simulink model "scdskyhogg"  (Simulink 7.6)
settings: Solver=ode45  StartTime=0.0  StopTime=75  RelTol=1e-3
model workspace (MAT data in the model file):
  cg_0 = [2.158 0 0]
  g_0 = [0 0 9.81]
  Sref = 20.9775
  bref = 12.5425
  cbar = 1.7526
  Thrust = 2512.574
  maxdef_aileron = 30
  mindef_aileron = -30
  maxdef_elevator = 20
  mindef_elevator = -20
  maxdef_rudder = 60
  mindef_rudder = -60
  wn_act = 44
  z_act = 0.7
  LatLong0 = [45 120]
  heading0 = 0
  Tc = 0.0166666666667
  mass = 1299.21378662
  inertia = [5787.969  0  117.64; 0  6928.93  0; -117.64  0  11578.329]
  Ts = 0
  alpha0 = 0.0170924
  V0 = 93.1047999839
  beta0 = 0
  alt0 = 2000
  wy0 = 0
  theta0 = 0.017092
  mpoperpoint : opcond.OperatingPoint (value not decoded)
  op : opcond.OperatingPoint (value not decoded)
  x0.time = 75
  x0.signals(1).values = 0
  x0.signals(1).dimensions = 1
  x0.signals(1).label = 'CSTATE'
  x0.signals(1).blockName = 'scdskyhogg/Environment/Wind Models/Discrete Wind Gust Model/Distance into
    | gust (x)/Distance into
    | Gust (x)
    | (Limited to gust length d)'
  x0.signals(1).stateName = ''
  x0.signals(1).inReferencedModel = 0
  x0.signals(1).sampleTime = [0 0]
  x0.signals(2).values = 0
  x0.signals(2).dimensions = 1
  x0.signals(2).label = 'CSTATE'
  x0.signals(2).blockName = 'scdskyhogg/Environment/Wind Models/Discrete Wind Gust Model/Distance into
    | gust (y)/Distance into
    | Gust (x)
    | (Limited to gust length d)
    | '
  x0.signals(2).stateName = ''
  x0.signals(2).inReferencedModel = 0
  x0.signals(2).sampleTime = [0 0]
  x0.signals(3).values = 0
  x0.signals(3).dimensions = 1
  x0.signals(3).label = 'CSTATE'
  x0.signals(3).blockName = 'scdskyhogg/Environment/Wind Models/Discrete Wind Gust Model/Distance into
    | gust (z)/Distance into
    | Gust (x)
    | (Limited to gust length d)
    | '
  x0.signals(3).stateName = ''
  x0.signals(3).inReferencedModel = 0
  x0.signals(3).sampleTime = [0 0]
  x0.signals(4).values = [0 0]
  x0.signals(4).dimensions = 2
  x0.signals(4).label = 'CSTATE'
  x0.signals(4).blockName = 'scdskyhogg/Environment/Wind Models/Dryden Wind Turbulence Model 
    | (Continuous (+q +r))/Filters on angular rates/Hpgw/pgw_p'
  x0.signals(4).stateName = ''
  x0.signals(4).inReferencedModel = 0
  x0.signals(4).sampleTime = [0 0]
  x0.signals(5).values = [0 0]
  x0.signals(5).dimensions = 2
  x0.signals(5).label = 'CSTATE'
  x0.signals(5).blockName = 'scdskyhogg/Environment/Wind Models/Dryden Wind Turbulence Model 
    | (Continuous (+q +r))/Filters on angular rates/Hqgw/qgw_p'
  x0.signals(5).stateName = ''
  x0.signals(5).inReferencedModel = 0
  x0.signals(5).sampleTime = [0 0]
  x0.signals(6).values = [0 0]
  x0.signals(6).dimensions = 2
  x0.signals(6).label = 'CSTATE'
  x0.signals(6).blockName = 'scdskyhogg/Environment/Wind Models/Dryden Wind Turbulence Model 
    | (Continuous (+q +r))/Filters on angular rates/Hrgw/rgw_p'
  x0.signals(6).stateName = ''
  x0.signals(6).inReferencedModel = 0
  x0.signals(6).sampleTime = [0 0]
  x0.signals(7).values = [0 0]
  x0.signals(7).dimensions = 2
  x0.signals(7).label = 'CSTATE'
  x0.signals(7).blockName = 'scdskyhogg/Environment/Wind Models/Dryden Wind Turbulence Model 
    | (Continuous (+q +r))/Filters on velocities/Hugw(s)/ug_p'
  x0.signals(7).stateName = ''
  x0.signals(7).inReferencedModel = 0
  x0.signals(7).sampleTime = [0 0]
  x0.signals(8).values = [0 0]
  x0.signals(8).dimensions = 2
  x0.signals(8).label = 'CSTATE'
  x0.signals(8).blockName = 'scdskyhogg/Environment/Wind Models/Dryden Wind Turbulence Model 
    | (Continuous (+q +r))/Filters on velocities/Hvgw(s)/vg_p1'
  x0.signals(8).stateName = ''
  x0.signals(8).inReferencedModel = 0
  x0.signals(8).sampleTime = [0 0]
  x0.signals(9).values = [0 0]
  x0.signals(9).dimensions = 2
  x0.signals(9).label = 'CSTATE'
  x0.signals(9).blockName = 'scdskyhogg/Environment/Wind Models/Dryden Wind Turbulence Model 
    | (Continuous (+q +r))/Filters on velocities/Hvgw(s)/vgw_p2'
  x0.signals(9).stateName = ''
  x0.signals(9).inReferencedModel = 0
  x0.signals(9).sampleTime = [0 0]
  x0.signals(10).values = [0 0]
  x0.signals(10).dimensions = 2
  x0.signals(10).label = 'CSTATE'
  x0.signals(10).blockName = 'scdskyhogg/Environment/Wind Models/Dryden Wind Turbulence Model 
    | (Continuous (+q +r))/Filters on velocities/Hwgw(s)/wg_p1'
  x0.signals(10).stateName = ''
  x0.signals(10).inReferencedModel = 0
  x0.signals(10).sampleTime = [0 0]
  x0.signals(11).values = [0 0]
  x0.signals(11).dimensions = 2
  x0.signals(11).label = 'CSTATE'
  x0.signals(11).blockName = 'scdskyhogg/Environment/Wind Models/Dryden Wind Turbulence Model 
    | (Continuous (+q +r))/Filters on velocities/Hwgw(s)/wg_p2'
  x0.signals(11).stateName = ''
  x0.signals(11).inReferencedModel = 0
  x0.signals(11).sampleTime = [0 0]
  x0.signals(12).values = 8000
  x0.signals(12).dimensions = 1
  x0.signals(12).label = 'CSTATE'
  x0.signals(12).blockName = 'scdskyhogg/Pilot/Transfer Fcn
    | (with initial outputs)/State Space'
  x0.signals(12).stateName = ''
  x0.signals(12).inReferencedModel = 0
  x0.signals(12).sampleTime = [0 0]
  x0.signals(13).values = [19554.3139246 18764.5538786]
  x0.signals(13).dimensions = 2
  x0.signals(13).label = 'DSTATE'
  x0.signals(13).blockName = 'scdskyhogg/Vehicle System Model/Avionics/Autopilot/Alt Controller'
  x0.signals(13).stateName = ''
  x0.signals(13).inReferencedModel = 0
  x0.signals(13).sampleTime = [0.0166666666667 0]
  x0.signals(14).values = 4.54490878098
  x0.signals(14).dimensions = 1
  x0.signals(14).label = 'DSTATE'
  x0.signals(14).blockName = 'scdskyhogg/Vehicle System Model/Avionics/Autopilot/Theta Controller'
  x0.signals(14).stateName = ''
  x0.signals(14).inReferencedModel = 0
  x0.signals(14).sampleTime = [0.0166666666667 0]
  x0.signals(15).values = [0 0]
  x0.signals(15).dimensions = 2
  x0.signals(15).label = 'DSTATE'
  x0.signals(15).blockName = 'scdskyhogg/Vehicle System Model/Avionics/Three-axis IMU/Three-axis Accelerometer/Dynamics/Second-order Dynamics/Transfer Fcn X/Discrete
    | Transfer Fcn'
  x0.signals(15).stateName = ''
  x0.signals(15).inReferencedModel = 0
  x0.signals(15).sampleTime = [0.0166666666667 0]
  x0.signals(16).values = [0 0]
  x0.signals(16).dimensions = 2
  x0.signals(16).label = 'DSTATE'
  x0.signals(16).blockName = 'scdskyhogg/Vehicle System Model/Avionics/Three-axis IMU/Three-axis Accelerometer/Dynamics/Second-order Dynamics/Transfer Fcn Y/Discrete
    | Transfer Fcn'
  x0.signals(16).stateName = ''
  x0.signals(16).inReferencedModel = 0
  x0.signals(16).sampleTime = [0.0166666666667 0]
  x0.signals(17).values = [0 0]
  x0.signals(17).dimensions = 2
  x0.signals(17).label = 'DSTATE'
  x0.signals(17).blockName = 'scdskyhogg/Vehicle System Model/Avionics/Three-axis IMU/Three-axis Accelerometer/Dynamics/Second-order Dynamics/Transfer Fcn Z/Discrete
    | Transfer Fcn'
  x0.signals(17).stateName = ''
  x0.signals(17).inReferencedModel = 0
  x0.signals(17).sampleTime = [0.0166666666667 0]
  x0.signals(18).values = [0 0]
  x0.signals(18).dimensions = 2
  x0.signals(18).label = 'DSTATE'
  x0.signals(18).blockName = 'scdskyhogg/Vehicle System Model/Avionics/Three-axis IMU/Three-axis Gyroscope/Dynamics/Second-order Dynamics/Transfer Fcn X/Discrete
    | Transfer Fcn'
  x0.signals(18).stateName = ''
  x0.signals(18).inReferencedModel = 0
  x0.signals(18).sampleTime = [0.0166666666667 0]
  x0.signals(19).values = [0 0]
  x0.signals(19).dimensions = 2
  x0.signals(19).label = 'DSTATE'
  x0.signals(19).blockName = 'scdskyhogg/Vehicle System Model/Avionics/Three-axis IMU/Three-axis Gyroscope/Dynamics/Second-order Dynamics/Transfer Fcn Y/Discrete
    | Transfer Fcn'
  x0.signals(19).stateName = ''
  x0.signals(19).inReferencedModel = 0
  x0.signals(19).sampleTime = [0.0166666666667 0]
  x0.signals(20).values = [0 0]
  x0.signals(20).dimensions = 2
  x0.signals(20).label = 'DSTATE'
  x0.signals(20).blockName = 'scdskyhogg/Vehicle System Model/Avionics/Three-axis IMU/Three-axis Gyroscope/Dynamics/Second-order Dynamics/Transfer Fcn Z/Discrete
    | Transfer Fcn'
  x0.signals(20).stateName = ''
  x0.signals(20).inReferencedModel = 0
  x0.signals(20).sampleTime = [0.0166666666667 0]
  x0.signals(21).values = [6983.69332589 -2000.01117817]
  x0.signals(21).dimensions = 2
  x0.signals(21).label = 'CSTATE'
  x0.signals(21).blockName = 'scdskyhogg/Vehicle System Model/Vehicle/3DoF to 6DoF/3DoF (Body Axes)/Position'
  x0.signals(21).stateName = ''
  x0.signals(21).inReferencedModel = 0
  x0.signals(21).sampleTime = [0 0]
  x0.signals(22).values = 0.0170954076892
  x0.signals(22).dimensions = 1
  x0.signals(22).label = 'CSTATE'
  x0.signals(22).blockName = 'scdskyhogg/Vehicle System Model/Vehicle/3DoF to 6DoF/3DoF (Body Axes)/Theta'
  x0.signals(22).stateName = ''
  x0.signals(22).inReferencedModel = 0
  x0.signals(22).sampleTime = [0 0]
  x0.signals(23).values = [93.0805745614 1.59150213219]
  x0.signals(23).dimensions = 2
  x0.signals(23).label = 'CSTATE'
  x0.signals(23).blockName = 'scdskyhogg/Vehicle System Model/Vehicle/3DoF to 6DoF/3DoF (Body Axes)/U,w'
  x0.signals(23).stateName = ''
  x0.signals(23).inReferencedModel = 0
  x0.signals(23).sampleTime = [0 0]
  x0.signals(24).values = -4.21452165535e-07
  x0.signals(24).dimensions = 1
  x0.signals(24).label = 'CSTATE'
  x0.signals(24).blockName = 'scdskyhogg/Vehicle System Model/Vehicle/3DoF to 6DoF/3DoF (Body Axes)/q'
  x0.signals(24).stateName = ''
  x0.signals(24).inReferencedModel = 0
  x0.signals(24).sampleTime = [0 0]
  x0.signals(25).values = 0
  x0.signals(25).dimensions = 1
  x0.signals(25).label = 'CSTATE'
  x0.signals(25).blockName = 'scdskyhogg/Vehicle System Model/Vehicle/AirframeActuators/2nd Order Non-linear Actuator/Limited
    | Deflection'
  x0.signals(25).stateName = ''
  x0.signals(25).inReferencedModel = 0
  x0.signals(25).sampleTime = [0 0]
  x0.signals(26).values = 0
  x0.signals(26).dimensions = 1
  x0.signals(26).label = 'CSTATE'
  x0.signals(26).blockName = 'scdskyhogg/Vehicle System Model/Vehicle/AirframeActuators/2nd Order Non-linear Actuator/Servo rate'
  x0.signals(26).stateName = ''
  x0.signals(26).inReferencedModel = 0
  x0.signals(26).sampleTime = [0 0]
  x0.signals(27).values = -0.905026907299
  x0.signals(27).dimensions = 1
  x0.signals(27).label = 'CSTATE'
  x0.signals(27).blockName = 'scdskyhogg/Vehicle System Model/Vehicle/AirframeActuators/2nd Order Non-linear Actuator1/Limited
    | Deflection'
  x0.signals(27).stateName = ''
  x0.signals(27).inReferencedModel = 0
  x0.signals(27).sampleTime = [0 0]
  x0.signals(28).values = 7.66583857879e-05
  x0.signals(28).dimensions = 1
  x0.signals(28).label = 'CSTATE'
  x0.signals(28).blockName = 'scdskyhogg/Vehicle System Model/Vehicle/AirframeActuators/2nd Order Non-linear Actuator1/Servo rate'
  x0.signals(28).stateName = ''
  x0.signals(28).inReferencedModel = 0
  x0.signals(28).sampleTime = [0 0]
  x0.signals(29).values = 0
  x0.signals(29).dimensions = 1
  x0.signals(29).label = 'CSTATE'
  x0.signals(29).blockName = 'scdskyhogg/Vehicle System Model/Vehicle/AirframeActuators/2nd Order Non-linear Actuator2/Limited
    | Deflection'
  x0.signals(29).stateName = ''
  x0.signals(29).inReferencedModel = 0
  x0.signals(29).sampleTime = [0 0]
  x0.signals(30).values = 0
  x0.signals(30).dimensions = 1
  x0.signals(30).label = 'CSTATE'
  x0.signals(30).blockName = 'scdskyhogg/Vehicle System Model/Vehicle/AirframeActuators/2nd Order Non-linear Actuator2/Servo rate'
  x0.signals(30).stateName = ''
  x0.signals(30).inReferencedModel = 0
  x0.signals(30).sampleTime = [0 0]
PreLoadFcn:
  | load asbSkyHoggData.mat
StartFcn:
  | warning('off','Simulink:blocks:BmathSqrtOfNegativeNumber');
  | warning('off','Simulink:Engine:UINotUpdatedDuringRapidAccelSim')
StopFcn:
  | warning('on','Simulink:blocks:BmathSqrtOfNegativeNumber');
values from neighbouring files (symbols this model uses):
  mass = 13.98/Kg2slug    (= 204.022661401)    [scd_aero_guid_dat.m]
  Tc = simout.time    [scdcompdelay_engspeed.m]
  Thrust = 10e3    (= 10000)    [scd_aero_guid_dat.m]
  Ts = 0.25    [scdcompdelay_engspeed.m]
undefined symbols (not defined in the file or in its folder): Earth, F, Light, MIL, statdyn, WGS84
libraries: aerolibasang x4, aerolibwind2 x3, aerolibtransform2 x3, aerolibactuator x3, aerolibatmos2 x2, aerolibobsolete x2, aerolibconvert2 x2, aerolibadyn x2, simulink x1, simulink_extras x1, aerolibnav x1, aerolib3dof2 x1
Description:
  | Lightweight Airplane Design
  | 
  | This is the three degree-of-freedom model of a lightweight four-seater
  | low wing monoplane with a longitudinal autopilot.
CloseFcn:
  | warning('on','Simulink:Engine:UINotUpdatedDuringRapidAccelSim')
settings Model: Creator=The MathWorks Inc.  SimulationMode=rapid-accelerator
settings DataIOCC: ExternalInput=[]  InitialState=x0  LoadExternalInput=on  LoadInitialState=on
settings OptimizationCC: InitFltsAndDblsToZero=on
settings DebuggingCC: AlgebraicLoopMsg=none  SaveWithParameterizedLinksMsg=none  SignalResolutionControl=TryResolveAllWithWarning  SolverPrmCheckMsg=none  UnconnectedInputMsg=none  UnconnectedOutputMsg=none  UnconnectedLineMsg=none  StrictBusMsg=Warning
settings GRTTargetCC: TargetFcnLib=ansi_tfl_tmw.mat

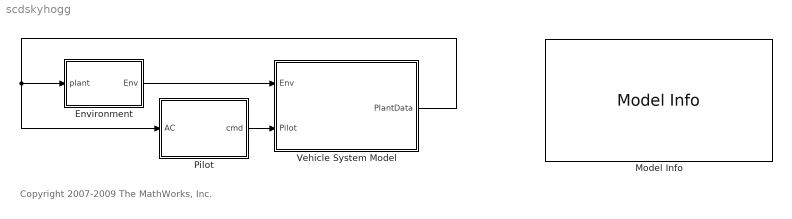
== system scdskyhogg ==
  note: Copyright 2007-2009 The MathWorks, Inc.
  Environment : Subsystem  TreatAsAtomicUnit=on
  Model Info : simulink/Model-Wide Utilities/Model Info  SystemSampleTime=-1  InitialBlockCM=None  BlockCM=None  Frame=on  DisplayStringWithTags=|  HorizontalTextAlignment=Center  LeftAlignmentValue=0.5  SourceBlockDiagram=scdskyhogg  TagMaxNumber=20
      | Sky Hogg demonstration model,
      | 
      | Vehicle Geometry from 
      | Cannon, M, Gabbard, M, Meyer, T, Morrison, 
      | S, Skocik, M, Woods, D. "Swineworks D-200 
      | Sky Hogg Design Proposal." AIAA/General 
      | Dynamics Corporation Team Aircraft Design
      |  Competition, 1991-1992
  Pilot : Subsystem  TreatAsAtomicUnit=on
  Vehicle System Model : Subsystem
      mask Display: image(imread('asbSkyHogg.jpg'),[.1 .1 .8 .8],'on')
  wires:
  Environment/1(Env) -> Vehicle System Model/1(Env)
  Vehicle System Model/1(PlantData) -> Environment/1(plant), Pilot/1(AC)
  Pilot/1(cmd) -> Vehicle System Model/2(Pilot)

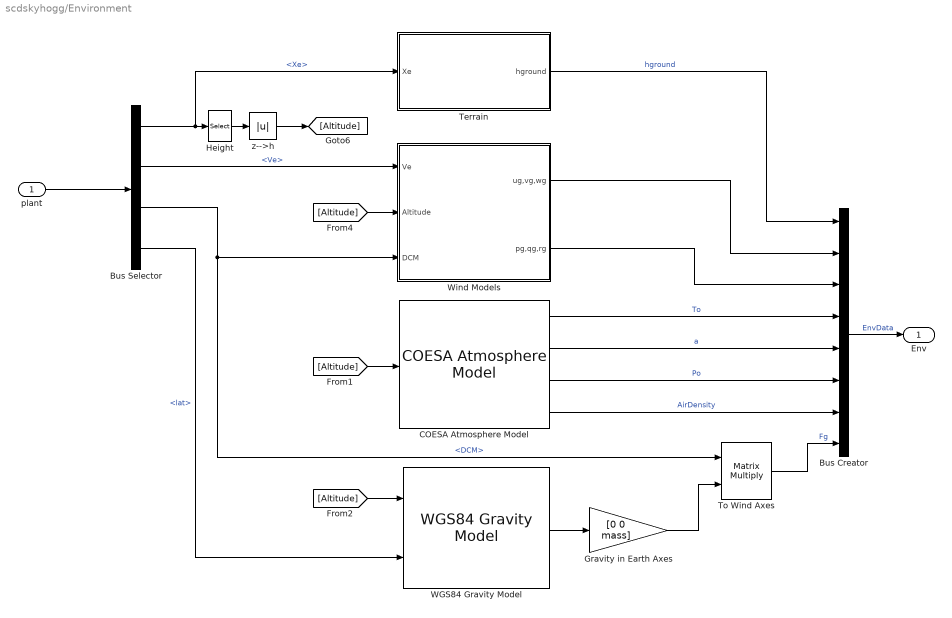
== system scdskyhogg/Environment ==
  plant : Inport
  Bus Creator : BusCreator  Inputs='hground','WindVelocity','WindAngularRates','To','a','Po','AirDensity','Fg'
  Bus Selector : BusSelector  OutputSignals=Xe,Ve,DCM,lat
  COESA Atmosphere Model : aerolibatmos2/COESA Atmosphere Model  SystemSampleTime=-1  units=Metric (MKS)  spec=1976 COESA-extended U.S. Standard Atmosphere  model=Profile  profile_var=High temperature  profile_percent=1%  profile_alt=5 km (16404 ft)  envelope_var=High temperature  envelope_percent=1%  action=Warning
  Gravity in Earth Axes : Gain  Gain=[0 0 mass]  SaturateOnIntegerOverflow=on  OutDataTypeStr=Inherit: Same as input  ParamDataTypeStr=Inherit: Same as input
  Height : Selector  InputPortWidth=3  IndexOptions=Index vector (dialog)  Indices=[3]  OutputSizes=1
  Terrain : Subsystem
  To Wind Axes : Product  Multiplication=Matrix(*)  SaturateOnIntegerOverflow=on  InputSameDT=on  OutDataTypeStr=Inherit: Same as first input
  WGS84 Gravity Model : aerolibobsolete/WGS84 Gravity Model  SystemSampleTime=-1  model=WGS84 Taylor Series  units=Metric (MKS)  no_atmos=on  precessing=on  month=February  day=1  year=2000  no_centrifugal=on  action=Warning
  Wind Models : Subsystem
  z-->h : Abs  SaturateOnIntegerOverflow=on
  Env : Outport  InitialOutput=0
  wires:
  Bus Selector/3 -> Wind Models/3(DCM), To Wind Axes/1  "<DCM>"
  Bus Selector/2 -> Wind Models/1(Ve)  "<Ve>"
  Bus Selector/1 -> Height/1, Terrain/1(Xe)  "<Xe>"
  [Altitude] -> COESA Atmosphere Model/1
  [Altitude] -> WGS84 Gravity Model/1
  [Altitude] -> Wind Models/2(Altitude)
  z-->h/1 -> [Altitude]
  plant/1 -> Bus Selector/1
  Bus Creator/1 -> Env/1  "EnvData"
  To Wind Axes/1 -> Bus Creator/8  "Fg"
  Gravity in Earth Axes/1 -> To Wind Axes/2
  WGS84 Gravity Model/1 -> Gravity in Earth Axes/1
  Bus Selector/4 -> WGS84 Gravity Model/2  "<lat>"
  Height/1 -> z-->h/1
  COESA Atmosphere Model/1 -> Bus Creator/4  "To"
  COESA Atmosphere Model/3 -> Bus Creator/6  "Po"
  COESA Atmosphere Model/2 -> Bus Creator/5  "a"
  COESA Atmosphere Model/4 -> Bus Creator/7  "AirDensity"
  Wind Models/2(pg,qg,rg) -> Bus Creator/3
  Wind Models/1(ug,vg,wg) -> Bus Creator/2
  Terrain/1(hground) -> Bus Creator/1  "hground"

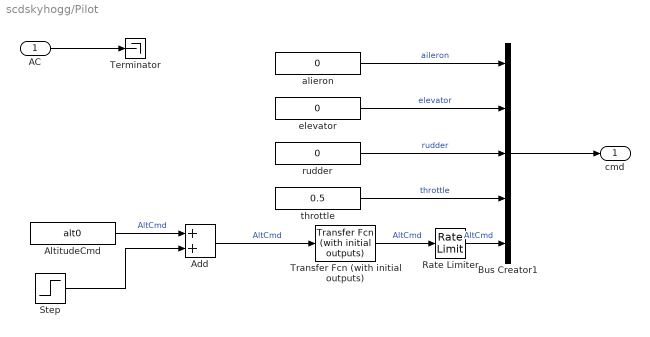
== system scdskyhogg/Pilot ==
  AC : Inport
  Add : Sum
  AltitudeCmd : Constant  Value=alt0  OutDataTypeStr=double
  Bus Creator1 : BusCreator  Inputs=5
  Rate Limiter : RateLimiter  RisingSlewLimit=500/3/60  SampleTimeMode=inherited  InitialCondition=2000
  Step : Step  Time=5  After=0  SampleTime=0
  Terminator : Terminator
  Transfer Fcn (with initial outputs) : simulink_extras/Additional Linear/Transfer Fcn (with initial outputs)  SystemSampleTime=-1  N=.25  D=[1,.25]  Y0=2000  U0=2000
  alieron : Constant  Value=0  OutDataTypeStr=single
  elevator : Constant  Value=0  OutDataTypeStr=single
  rudder : Constant  Value=0  OutDataTypeStr=single
  throttle : Constant  Value=0.5  OutDataTypeStr=double
  cmd : Outport
  wires:
  elevator/1 -> Bus Creator1/2  "elevator"
  alieron/1 -> Bus Creator1/1  "aileron"
  throttle/1 -> Bus Creator1/4  "throttle"
  rudder/1 -> Bus Creator1/3  "rudder"
  Bus Creator1/1 -> cmd/1
  AC/1 -> Terminator/1
  AltitudeCmd/1 -> Add/1  "AltCmd"
  Step/1 -> Add/2
  Add/1 -> Transfer Fcn (with initial outputs)/1  "AltCmd"
  Rate Limiter/1 -> Bus Creator1/5  "AltCmd"
  Transfer Fcn (with initial outputs)/1 -> Rate Limiter/1  "AltCmd"

== system scdskyhogg/Vehicle System Model ==
  Env : Inport
  Pilot : Inport  Port=2
  Avionics : Subsystem
  "Env " : InportShadow  Port=1
  Flight Sensors : Subsystem
  "Pilot " : InportShadow  Port=2
  Vehicle : Subsystem
  PlantData : Outport
  wires:
  Env/1 -> Vehicle/1(Env)
  Vehicle/1(PlantData) -> Avionics/1(PlantData), Flight Sensors/2(plant), PlantData/1
  Flight Sensors/1(sensed) -> Avionics/2(Sensors)
  Avionics/1(ActCmd) -> Vehicle/2(ActCmd)
  Pilot/1 -> Vehicle/3(Pilot)
  "Env "/1 -> Flight Sensors/1(Env)
  "Pilot "/1 -> Avionics/3(Pilot)

== system scdskyhogg/Environment/Terrain ==
  note: This part of the system defines the interface for the terrain model that will be developed in detail later on.
  Xe : Inport
  Terminator : Terminator
  hground_value : Constant  Value=0  OutDataTypeStr=single
  hground : Outport
  wires:
  hground_value/1 -> hground/1  "hground"
  Xe/1 -> Terminator/1

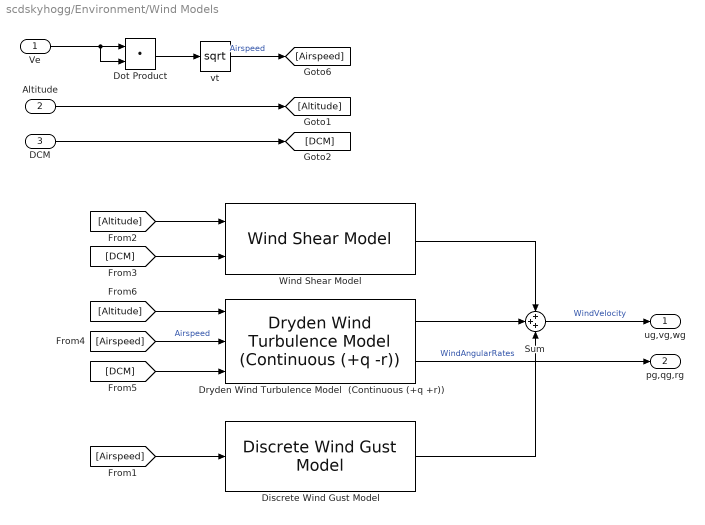
== system scdskyhogg/Environment/Wind Models ==
  Ve : Inport
  Altitude : Inport  Port=2
  DCM : Inport  Port=3
  Discrete Wind Gust Model : aerolibwind2/Discrete Wind Gust Model  SystemSampleTime=-1  units=Metric (MKS)  Gx=off  Gy=off  Gz=off  t_0=20  d_m=[120 120 80]  v_m=[3.5 3.0 3.0]
  Dot Product : DotProduct  OutDataTypeStr=Inherit: Inherit via internal rule
  Dryden Wind Turbulence Model  (Continuous (+q +r)) : aerolibwind2/Dryden Wind Turbulence Model  (Continuous (+q -r))  SystemSampleTime=-1  units=Metric (MKS)  spec=MIL-F-8785C  model=Continuous Dryden (+q +r)  W20=5  Wdeg=0  TurbProb=10^-2 - Light  L_high=533.4  Wingspan=4  ts=0.1  Seed=[23341 23342 23343 23344]  T_on=off
  Sum : Sum  Inputs=+++  SaturateOnIntegerOverflow=on  InputSameDT=on  OutDataTypeStr=Inherit: Same as first input
  Wind Shear Model : aerolibwind2/Wind Shear Model  SystemSampleTime=-1  units=Metric (MKS)  phase=Category C - Terminal Flight Phase  W_20=1  Wdeg=0
  vt : Math  Operator=sqrt  SaturateOnIntegerOverflow=on
  ug,vg,wg : Outport
  pg,qg,rg : Outport  Port=2
  wires:
  [Altitude] -> Dryden Wind Turbulence Model  (Continuous (+q +r))/1
  [DCM] -> Dryden Wind Turbulence Model  (Continuous (+q +r))/3
  [DCM] -> Wind Shear Model/2
  DCM/1 -> [DCM]
  [Altitude] -> Wind Shear Model/1
  Altitude/1 -> [Altitude]
  [Airspeed] -> Discrete Wind Gust Model/1
  vt/1 -> [Airspeed]  "Airspeed"
  Dot Product/1 -> vt/1
  Dryden Wind Turbulence Model  (Continuous (+q +r))/2 -> pg,qg,rg/1  "WindAngularRates"
  [Airspeed] -> Dryden Wind Turbulence Model  (Continuous (+q +r))/2  "Airspeed"
  Sum/1 -> ug,vg,wg/1  "WindVelocity"
  Discrete Wind Gust Model/1 -> Sum/3
  Dryden Wind Turbulence Model  (Continuous (+q +r))/1 -> Sum/2
  Wind Shear Model/1 -> Sum/1
  Ve/1 -> Dot Product/2, Dot Product/1

== system scdskyhogg/Vehicle System Model/Avionics ==
  PlantData : Inport
  Sensors : Inport  Port=2
  Pilot : Inport  Port=3
  Air Data Computer : Subsystem  TreatAsAtomicUnit=on
  Autopilot : Subsystem
  Bus Creator : BusCreator  Inputs=2
  Bus Selector1 : BusSelector  OutputSignals=Ab,w,wdot
  Center of Gravity : Constant  Value=cg_0  SampleTime=Tc
  Gravity (not in Accels) : Constant  Value=g_0  SampleTime=Tc
  Guidance : Subsystem
  Three-axis IMU : aerolibnav/Three-axis Inertial Measurement Unit  SystemSampleTime=-1  units=Metric (MKS)  imu=cg_0  dtype_a=off  w_a=190  z_a=0.707  a_sf_cc=[1 0 0; 0 1 0; 0 0 1]  a_bias=[0 0 0]  a_sat="[-inf  -inf  -inf  inf inf inf]"  dtype_g=off  w_g=190  z_g=0.707  g_sf_cc=[1 0 0; 0 1 0; 0 0 1]  g_bias=[0 0 0]  g_sens=[0 0 0]  g_sat="[-inf  -inf  -inf  inf inf inf]"  i_rand=off  i_seeds=[23093 23094 23095 23096 23097 23098]  i_pow=[0.001 0.001 0.001 0.0001 0.0001 0.0001]  i_Ts=Tc
  ActCmd : Outport
  wires:
  Three-axis IMU/2 -> Bus Creator/2
  Three-axis IMU/1 -> Bus Creator/1
  Bus Selector1/1 -> Three-axis IMU/1  "<Ab>"
  Center of Gravity/1 -> Three-axis IMU/4
  Bus Creator/1 -> Guidance/2(AvionicBus), Autopilot/1(AvionicBus)
  PlantData/1 -> Bus Selector1/1
  Bus Selector1/2 -> Three-axis IMU/2  "<w>"
  Bus Selector1/3 -> Three-axis IMU/3  "<wdot>"
  Gravity (not in Accels)/1 -> Three-axis IMU/5
  Sensors/1 -> Air Data Computer/1(sensors)
  Autopilot/1(cmd) -> ActCmd/1
  Air Data Computer/1(AirData) -> Guidance/1(AirData), Autopilot/2(AirData)
  Guidance/1(cmd) -> Autopilot/3(guidance)
  Pilot/1 -> Guidance/3(Pilot)

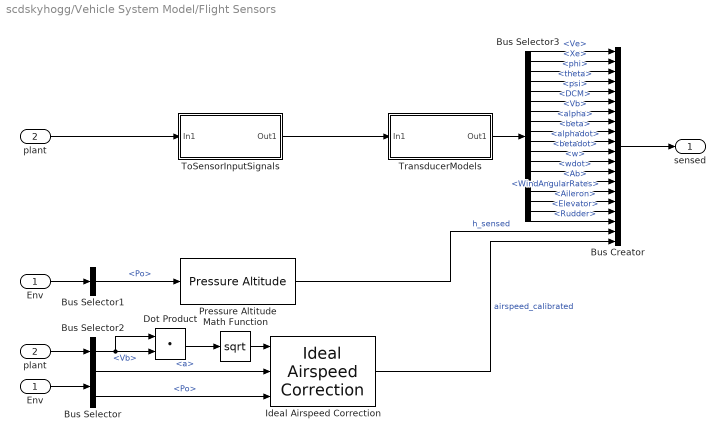
== system scdskyhogg/Vehicle System Model/Flight Sensors ==
  Env : Inport
  plant : Inport  Port=2
  Bus Creator : BusCreator  Inputs=20
  Bus Selector : BusSelector  OutputSignals=a,Po
  Bus Selector1 : BusSelector  OutputSignals=Po
  Bus Selector2 : BusSelector  OutputSignals=Vb
  Bus Selector3 : BusSelector  OutputSignals=Ve,Xe,body angles.phi,body angles.theta,body angles.psi,DCM,Vb,alpha,beta,alphadot,betadot,w,wdot,Ab,WindAngularRates,Act_positions.Aileron,Act_positions.Elevator,Act_positions.Rudder
  Dot Product : DotProduct  InputSameDT=on  OutDataTypeStr=Inherit: Inherit via internal rule
  "Env " : InportShadow  Port=1
  Ideal Airspeed Correction : aerolibasang/Ideal Airspeed Correction  SystemSampleTime=-1  units=Metric (MKS)  vel_in=TAS  vel_out_tas=CAS  vel_out_eas=CAS  vel_out_cas=TAS  action=Error
  Math Function : Math  Operator=sqrt  SaturateOnIntegerOverflow=on
  Pressure Altitude : aerolibatmos2/Pressure Altitude  SystemSampleTime=-1  units=Metric (MKS)  action=Warning
  ToSensorInputSignals : Subsystem
  TransducerModels : Subsystem
  "plant " : InportShadow  Port=2
  sensed : Outport
  wires:
  ToSensorInputSignals/1(Out1) -> TransducerModels/1(In1)
  Env/1 -> Bus Selector/1
  TransducerModels/1(Out1) -> Bus Selector3/1
  plant/1 -> ToSensorInputSignals/1(In1)
  Bus Selector/1 -> Ideal Airspeed Correction/2  "<a>"
  Bus Selector/2 -> Ideal Airspeed Correction/3  "<Po>"
  Bus Selector1/1 -> Pressure Altitude/1  "<Po>"
  "Env "/1 -> Bus Selector1/1
  "plant "/1 -> Bus Selector2/1
  Dot Product/1 -> Math Function/1
  Math Function/1 -> Ideal Airspeed Correction/1
  Bus Selector2/1 -> Dot Product/2, Dot Product/1  "<Vb>"
  Bus Selector3/1 -> Bus Creator/1  "<Ve>"
  Bus Selector3/2 -> Bus Creator/2  "<Xe>"
  Bus Selector3/3 -> Bus Creator/3  "<phi>"
  Bus Selector3/4 -> Bus Creator/4  "<theta>"
  Bus Selector3/5 -> Bus Creator/5  "<psi>"
  Bus Selector3/6 -> Bus Creator/6  "<DCM>"
  Bus Selector3/7 -> Bus Creator/7  "<Vb>"
  Bus Selector3/8 -> Bus Creator/8  "<alpha>"
  Bus Selector3/9 -> Bus Creator/9  "<beta>"
  Bus Selector3/10 -> Bus Creator/10  "<alphadot>"
  Bus Selector3/11 -> Bus Creator/11  "<betadot>"
  Bus Selector3/12 -> Bus Creator/12  "<w>"
  Bus Selector3/13 -> Bus Creator/13  "<wdot>"
  Bus Selector3/14 -> Bus Creator/14  "<Ab>"
  Bus Creator/1 -> sensed/1
  Bus Selector3/15 -> Bus Creator/15  "<WindAngularRates>"
  Bus Selector3/16 -> Bus Creator/16  "<Aileron>"
  Bus Selector3/17 -> Bus Creator/17  "<Elevator>"
  Bus Selector3/18 -> Bus Creator/18  "<Rudder>"
  Pressure Altitude/1 -> Bus Creator/19  "h_sensed"
  Ideal Airspeed Correction/1 -> Bus Creator/20  "airspeed_calibrated"

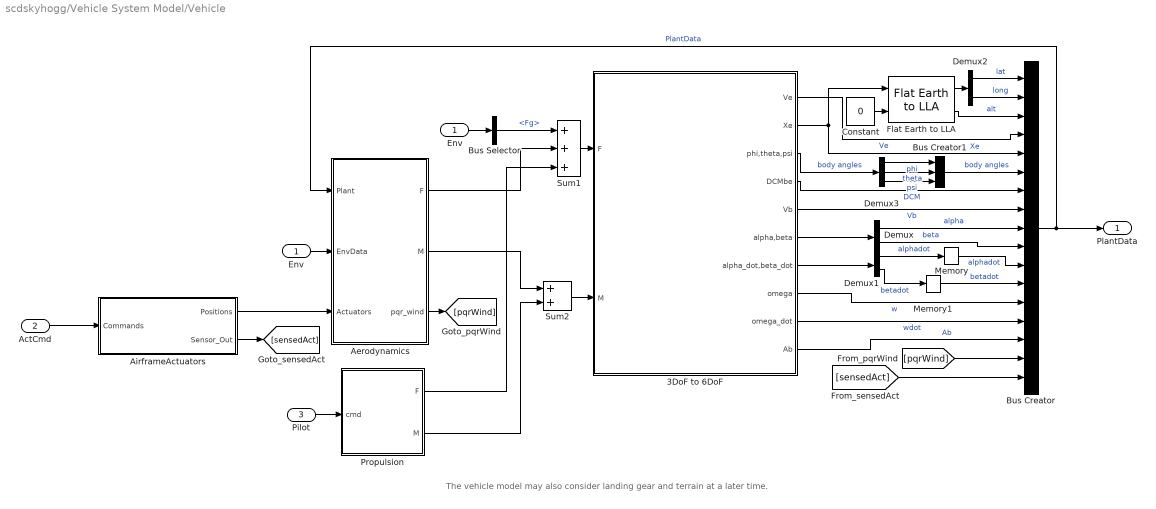
== system scdskyhogg/Vehicle System Model/Vehicle ==
  note: The vehicle model may also consider landing gear and terrain at a later time.
  Env : Inport
  ActCmd : Inport  Port=2
  Pilot : Inport  Port=3
  3DoF to 6DoF : Subsystem
  Aerodynamics : Subsystem
  AirframeActuators : Subsystem
  Bus Creator : BusCreator  Inputs=17
  Bus Creator1 : BusCreator  Inputs=3
  Bus Selector : BusSelector  OutputSignals=Fg
  Constant : Constant  Value=0
  Demux : Demux  Outputs=2
  Demux1 : Demux  Outputs=2
  Demux2 : Demux  Outputs=2
  Demux3 : Demux  Outputs=3
  "Env " : InportShadow  Port=1
  Flat Earth to LLA : aerolibtransform2/Flat Earth to LLA  SystemSampleTime=-1  units=Metric (MKS)  ptype=Earth (WGS84)  F=1/298.257223563  R=6378137  LL0=LatLong0  psi=heading0
  Memory : Memory  X0=alpha0  LinearizeMemory=on
  Memory1 : Memory  X0=beta0  LinearizeMemory=on
  Propulsion : Subsystem
      settings: RTWSystemCode=Inline
  Sum1 : Sum  Inputs=+++  SaturateOnIntegerOverflow=on  InputSameDT=on  OutDataTypeStr=Inherit: Same as first input
  Sum2 : Sum  SaturateOnIntegerOverflow=on  InputSameDT=on  OutDataTypeStr=Inherit: Same as first input
  PlantData : Outport
  wires:
  Sum1/1 -> 3DoF to 6DoF/1(F)
  Sum2/1 -> 3DoF to 6DoF/2(M)
  3DoF to 6DoF/3(phi,theta,psi) -> Demux3/1  "body angles"
  3DoF to 6DoF/4(DCMbe) -> Bus Creator/7  "DCM"
  3DoF to 6DoF/5(Vb) -> Bus Creator/8  "Vb"
  3DoF to 6DoF/6(alpha,beta) -> Demux/1
  3DoF to 6DoF/7(alpha_dot,beta_dot) -> Demux1/1
  3DoF to 6DoF/9(omega_dot) -> Bus Creator/14  "wdot"
  3DoF to 6DoF/10(Ab) -> Bus Creator/15  "Ab"
  Bus Creator/1 -> Aerodynamics/1(Plant), PlantData/1  "PlantData"
  Aerodynamics/1(F) -> Sum1/2
  Aerodynamics/2(M) -> Sum2/1
  Propulsion/1(F) -> Sum1/3
  Propulsion/2(M) -> Sum2/2
  Bus Selector/1 -> Sum1/1  "<Fg>"
  Env/1 -> Aerodynamics/2(EnvData)
  ActCmd/1 -> AirframeActuators/1(Commands)
  Pilot/1 -> Propulsion/1(cmd)
  "Env "/1 -> Bus Selector/1
  AirframeActuators/1(Positions) -> Aerodynamics/3(Actuators)
  Aerodynamics/3(pqr_wind) -> [pqrWind]
  [pqrWind] -> Bus Creator/16
  AirframeActuators/2(Sensor_Out) -> [sensedAct]
  [sensedAct] -> Bus Creator/17
  Constant/1 -> Flat Earth to LLA/2
  Flat Earth to LLA/2 -> Bus Creator/3  "alt"
  Flat Earth to LLA/1 -> Demux2/1
  Demux2/1 -> Bus Creator/1  "lat"
  Demux2/2 -> Bus Creator/2  "long"
  Demux1/1 -> Memory/1  "alphadot"
  Demux1/2 -> Memory1/1  "betadot"
  Demux3/1 -> Bus Creator1/1  "phi"
  Demux3/2 -> Bus Creator1/2  "theta"
  Demux3/3 -> Bus Creator1/3  "psi"
  Bus Creator1/1 -> Bus Creator/6  "body angles"
  3DoF to 6DoF/8(omega) -> Bus Creator/13  "w"
  Demux/2 -> Bus Creator/10  "beta"
  Demux/1 -> Bus Creator/9  "alpha"
  Memory/1 -> Bus Creator/11  "alphadot"
  Memory1/1 -> Bus Creator/12  "betadot"
  3DoF to 6DoF/1(Ve) -> Bus Creator/4  "Ve"
  3DoF to 6DoF/2(Xe) -> Flat Earth to LLA/1, Bus Creator/5  "Xe"

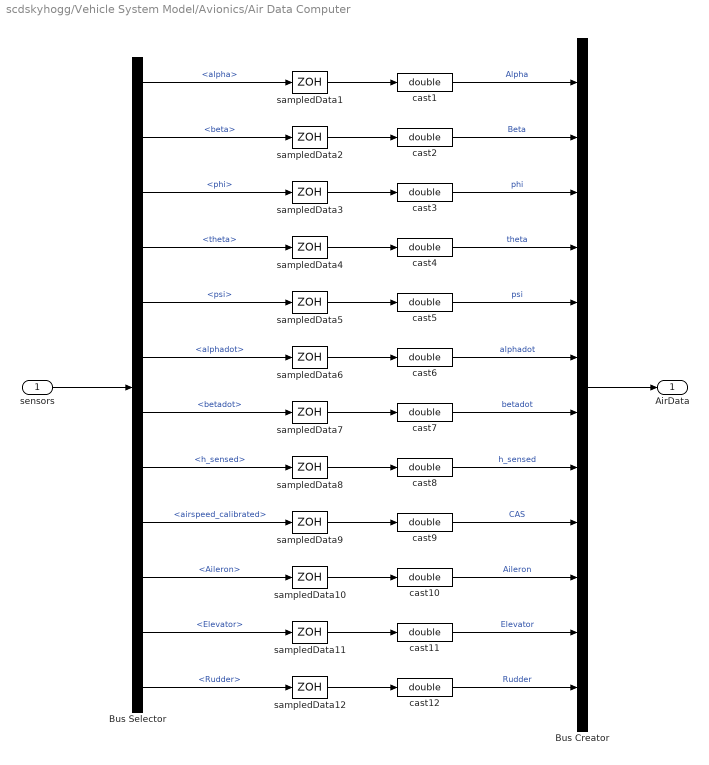
== system scdskyhogg/Vehicle System Model/Avionics/Air Data Computer ==
  sensors : Inport  SampleTime=Ts
  Bus Creator : BusCreator  Inputs=12
  Bus Selector : BusSelector  OutputSignals=alpha,beta,phi,theta,psi,alphadot,betadot,h_sensed,airspeed_calibrated,Aileron,Elevator,Rudder
  cast{1..12} (12 alike) : DataTypeConversion  OutDataTypeStr=double
  sampledData{1..12} (12 alike) : ZeroOrderHold  SampleTime=Tc
  AirData : Outport
  wires:
  sensors/1 -> Bus Selector/1
  Bus Creator/1 -> AirData/1
  cast1/1 -> Bus Creator/1  "Alpha"
  cast2/1 -> Bus Creator/2  "Beta"
  cast3/1 -> Bus Creator/3  "phi"
  cast12/1 -> Bus Creator/12  "Rudder"
  cast10/1 -> Bus Creator/10  "Aileron"
  cast9/1 -> Bus Creator/9  "CAS"
  cast8/1 -> Bus Creator/8  "h_sensed"
  cast7/1 -> Bus Creator/7  "betadot"
  cast6/1 -> Bus Creator/6  "alphadot"
  cast5/1 -> Bus Creator/5  "psi"
  sampledData1/1 -> cast1/1
  sampledData2/1 -> cast2/1
  sampledData3/1 -> cast3/1
  sampledData4/1 -> cast4/1
  sampledData5/1 -> cast5/1
  sampledData6/1 -> cast6/1
  sampledData7/1 -> cast7/1
  sampledData8/1 -> cast8/1
  sampledData9/1 -> cast9/1
  sampledData10/1 -> cast10/1
  cast4/1 -> Bus Creator/4  "theta"
  Bus Selector/1 -> sampledData1/1  "<alpha>"
  Bus Selector/2 -> sampledData2/1  "<beta>"
  Bus Selector/3 -> sampledData3/1  "<phi>"
  Bus Selector/4 -> sampledData4/1  "<theta>"
  Bus Selector/5 -> sampledData5/1  "<psi>"
  Bus Selector/6 -> sampledData6/1  "<alphadot>"
  Bus Selector/7 -> sampledData7/1  "<betadot>"
  Bus Selector/8 -> sampledData8/1  "<h_sensed>"
  Bus Selector/9 -> sampledData9/1  "<airspeed_calibrated>"
  Bus Selector/10 -> sampledData10/1  "<Aileron>"
  Bus Selector/12 -> sampledData12/1  "<Rudder>"
  sampledData11/1 -> cast11/1
  sampledData12/1 -> cast12/1
  Bus Selector/11 -> sampledData11/1  "<Elevator>"
  cast11/1 -> Bus Creator/11  "Elevator"

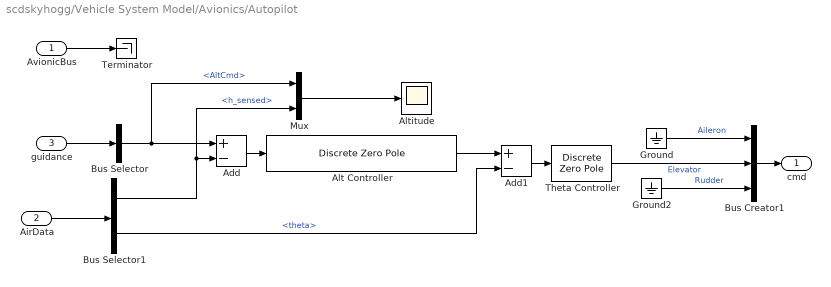
== system scdskyhogg/Vehicle System Model/Avionics/Autopilot ==
  AvionicBus : Inport
  AirData : Inport  Port=2
  guidance : Inport  Port=3
  Add : Sum  Inputs=+-
  Add1 : Sum  Inputs=+-
  Alt Controller : DiscreteZeroPole  Zeros=[0.998853192323097;0.977076159863424]  Poles=[1;0.920841826994512]  Gain=0.0337283240400683  SampleTime=Tc
  Altitude : Scope
      settings: TimeRange=75  YMin=2000  YMax=2060  Decimation=5
  Bus Creator1 : BusCreator  Inputs=3
  Bus Selector : BusSelector  OutputSignals=AltCmd
  Bus Selector1 : BusSelector  OutputSignals=h_sensed,theta
  Ground : Ground
  Ground2 : Ground
  Mux : Mux  Inputs=2
  Terminator : Terminator
  Theta Controller : DiscreteZeroPole  Zeros=0.999268009521977  Poles=1  Gain=-261.8699347622  SampleTime=Tc
  cmd : Outport
  wires:
  Add1/1 -> Theta Controller/1
  Alt Controller/1 -> Add1/1
  Add/1 -> Alt Controller/1
  Bus Selector/1 -> Mux/1, Add/1  "<AltCmd>"
  guidance/1 -> Bus Selector/1
  AirData/1 -> Bus Selector1/1
  AvionicBus/1 -> Terminator/1
  Bus Creator1/1 -> cmd/1
  Ground2/1 -> Bus Creator1/3  "Rudder"
  Theta Controller/1 -> Bus Creator1/2  "Elevator"
  Ground/1 -> Bus Creator1/1  "Aileron"
  Mux/1 -> Altitude/1
  Bus Selector1/1 -> Mux/2, Add/2  "<h_sensed>"
  Bus Selector1/2 -> Add1/2  "<theta>"

== system scdskyhogg/Vehicle System Model/Avionics/Guidance ==
  note: This part of the system defines the interface for the guidance model that will be developed in detail later on.
  AirData : Inport
  AvionicBus : Inport  Port=2
  Pilot : Inport  Port=3
  Bus Creator1 : BusCreator  Inputs=2
  Bus Selector : BusSelector  OutputSignals=AltCmd
  Ground1 : Ground
  Terminator : Terminator
  Terminator1 : Terminator
  cmd : Outport
  wires:
  Pilot/1 -> Bus Selector/1
  Bus Selector/1 -> Bus Creator1/1  "<AltCmd>"
  Ground1/1 -> Bus Creator1/2  "Elevator angle"
  Bus Creator1/1 -> cmd/1
  AvionicBus/1 -> Terminator/1
  AirData/1 -> Terminator1/1

== system scdskyhogg/Vehicle System Model/Flight Sensors/ToSensorInputSignals ==
  note: This part of the system defines the interface for the measurement noise model that
      |  will be developed in detail later on.
  In1 : Inport
  Out1 : Outport
  wires:
  In1/1 -> Out1/1

== system scdskyhogg/Vehicle System Model/Flight Sensors/TransducerModels ==
  note: This part of the system defines the interface for the transducers model that
      |  will be developed in detail later on.
  In1 : Inport
  Out1 : Outport
  wires:
  In1/1 -> Out1/1

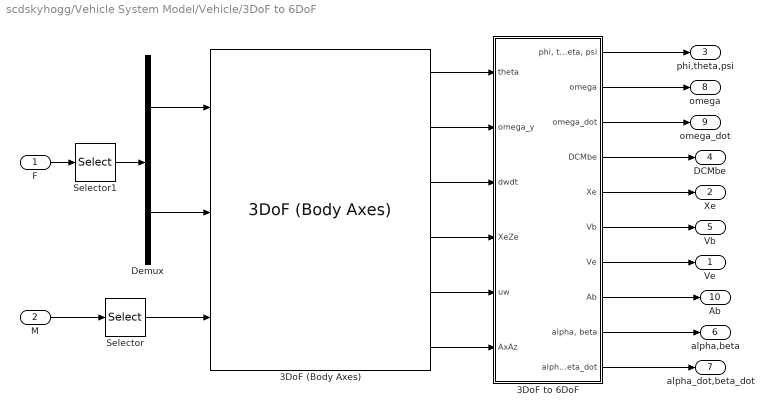
== system scdskyhogg/Vehicle System Model/Vehicle/3DoF to 6DoF ==
  F : Inport
  M : Inport  Port=2
  3DoF (Body Axes) : aerolib3dof2/3DoF (Body Axes)  SystemSampleTime=-1  units=Metric (MKS)  mtype=Fixed  v_ini=V0  theta_ini=theta0  alpha_ini=alpha0  q_ini=wy0  pos_ini=[0 -alt0]  mass=mass  mass_e=0.5  mass_f=3.0  Iyy=inertia(2,2)  Iyy_e=0.5  Iyy_f=3.0  g_in=Internal  g=0
  3DoF to 6DoF : Subsystem
  Demux : Demux  Outputs=2
  Selector : Selector  InputPortWidth=3  IndexOptions=Index vector (dialog)  Indices=2  OutputSizes=1
  Selector1 : Selector  InputPortWidth=3  IndexOptions=Index vector (dialog)  Indices=[1 3]  OutputSizes=1
  Ve : Outport
  Xe : Outport  Port=2
  phi,theta,psi : Outport  Port=3
  DCMbe : Outport  Port=4
  Vb : Outport  Port=5
  alpha,beta : Outport  Port=6
  alpha_dot,beta_dot : Outport  Port=7
  omega : Outport  Port=8
  omega_dot : Outport  Port=9
  Ab : Outport  Port=10
  wires:
  3DoF (Body Axes)/1 -> 3DoF to 6DoF/1(theta)
  F/1 -> Selector1/1
  M/1 -> Selector/1
  Selector/1 -> 3DoF (Body Axes)/3
  Selector1/1 -> Demux/1
  3DoF to 6DoF/2(omega) -> omega/1
  3DoF to 6DoF/3(omega_dot) -> omega_dot/1
  3DoF to 6DoF/5(Xe) -> Xe/1
  3DoF to 6DoF/7(Ve) -> Ve/1
  3DoF to 6DoF/10("alpha_dot, beta_dot") -> alpha_dot,beta_dot/1
  3DoF to 6DoF/1("phi, theta, psi") -> phi,theta,psi/1
  3DoF (Body Axes)/2 -> 3DoF to 6DoF/2(omega_y)
  3DoF to 6DoF/6(Vb) -> Vb/1
  3DoF to 6DoF/8(Ab) -> Ab/1
  3DoF to 6DoF/9("alpha, beta") -> alpha,beta/1
  3DoF to 6DoF/4(DCMbe) -> DCMbe/1
  3DoF (Body Axes)/3 -> 3DoF to 6DoF/3(dwdt)
  3DoF (Body Axes)/4 -> 3DoF to 6DoF/4(XeZe)
  3DoF (Body Axes)/5 -> 3DoF to 6DoF/5(uw)
  3DoF (Body Axes)/6 -> 3DoF to 6DoF/6(AxAz)
  Demux/1 -> 3DoF (Body Axes)/1
  Demux/2 -> 3DoF (Body Axes)/2

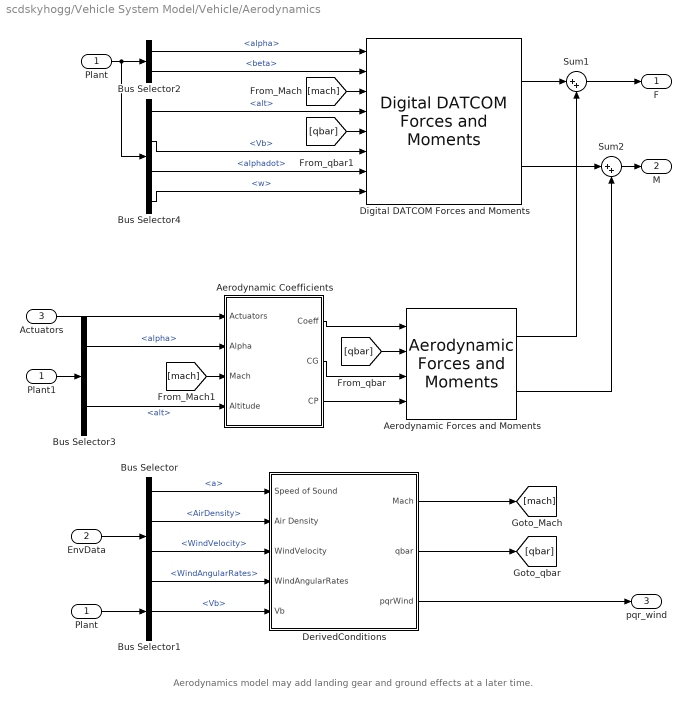
== system scdskyhogg/Vehicle System Model/Vehicle/Aerodynamics ==
  note: Aerodynamics model may add landing gear and ground effects at a later time.
  Plant : Inport
  EnvData : Inport  Port=2
  Actuators : Inport  Port=3
  Aerodynamic Coefficients : Subsystem
  "Aerodynamic Forces and Moments " : aerolibadyn/Aerodynamic Forces and Moments   SystemSampleTime=-1  inputAxes=Body  outputForceAxes=Body  outputMomentAxes=Body  S=Sref  b=bref  cbar=cbar
  Bus Selector : BusSelector  OutputSignals=a,AirDensity,WindVelocity,WindAngularRates
  Bus Selector1 : BusSelector  OutputSignals=Vb
  Bus Selector2 : BusSelector  OutputSignals=alpha,beta
  Bus Selector3 : BusSelector  OutputSignals=alpha,alt
  Bus Selector4 : BusSelector  OutputSignals=alt,Vb,alphadot,w
  DerivedConditions : Subsystem
  Digital DATCOM Forces and Moments : aerolibadyn/Digital DATCOM Forces and Moments  SystemSampleTime=-1  units=Metric (MKS)  dcase=statdyn{1}  fmode=Body  buildno=0  imethod=Linear  emethod=Linear  rmethod=Linear Extrapolation  action=None
  "Plant " : InportShadow  Port=1
  Plant1 : InportShadow  Port=1
  Sum1 : Sum  Inputs=|++
  Sum2 : Sum  Inputs=|++
  F : Outport
  M : Outport  Port=2
  pqr_wind : Outport  Port=3
  wires:
  Digital DATCOM Forces and Moments/1 -> Sum1/1
  Digital DATCOM Forces and Moments/2 -> Sum2/1
  Aerodynamic Coefficients/1(Coeff) -> "Aerodynamic Forces and Moments "/1
  Sum1/1 -> F/1
  "Aerodynamic Forces and Moments "/1 -> Sum1/2
  Sum2/1 -> M/1
  "Aerodynamic Forces and Moments "/2 -> Sum2/2
  EnvData/1 -> Bus Selector/1
  Bus Selector/1 -> DerivedConditions/1(Speed of Sound)  "<a>"
  Bus Selector/2 -> DerivedConditions/2(Air Density)  "<AirDensity>"
  Bus Selector/3 -> DerivedConditions/3(WindVelocity)  "<WindVelocity>"
  Bus Selector/4 -> DerivedConditions/4(WindAngularRates)  "<WindAngularRates>"
  "Plant "/1 -> Bus Selector1/1
  Bus Selector1/1 -> DerivedConditions/5(Vb)  "<Vb>"
  Plant/1 -> Bus Selector2/1, Bus Selector4/1
  Bus Selector2/1 -> Digital DATCOM Forces and Moments/1  "<alpha>"
  Bus Selector2/2 -> Digital DATCOM Forces and Moments/2  "<beta>"
  Plant1/1 -> Bus Selector3/1
  Bus Selector3/1 -> Aerodynamic Coefficients/2(Alpha)  "<alpha>"
  DerivedConditions/1(Mach) -> [mach]
  [mach] -> Digital DATCOM Forces and Moments/3
  Aerodynamic Coefficients/2(CG) -> "Aerodynamic Forces and Moments "/3
  Aerodynamic Coefficients/3(CP) -> "Aerodynamic Forces and Moments "/4
  DerivedConditions/2(qbar) -> [qbar]
  [qbar] -> "Aerodynamic Forces and Moments "/2
  [qbar] -> Digital DATCOM Forces and Moments/5
  Bus Selector4/2 -> Digital DATCOM Forces and Moments/6  "<Vb>"
  Bus Selector4/1 -> Digital DATCOM Forces and Moments/4  "<alt>"
  DerivedConditions/3("pqrWind ") -> pqr_wind/1
  Bus Selector4/3 -> Digital DATCOM Forces and Moments/7  "<alphadot>"
  Bus Selector4/4 -> Digital DATCOM Forces and Moments/8  "<w>"
  Actuators/1 -> Aerodynamic Coefficients/1(Actuators)
  Bus Selector3/2 -> Aerodynamic Coefficients/4(Altitude)  "<alt>"
  [mach] -> Aerodynamic Coefficients/3(Mach)

== system scdskyhogg/Vehicle System Model/Vehicle/AirframeActuators ==
  Commands : Inport
  2nd Order Non-linear Actuator : aerolibactuator/Second Order Nonlinear Actuator  SystemSampleTime=-1  wn_fin=wn_act  z_fin=z_act  fin_max=maxdef_aileron  fin_min=mindef_aileron  fin_maxrate=Inf  fin_act_0=0
  2nd Order Non-linear Actuator1 : aerolibactuator/Second Order Nonlinear Actuator  SystemSampleTime=-1  wn_fin=wn_act  z_fin=z_act  fin_max=maxdef_elevator  fin_min=mindef_elevator  fin_maxrate=Inf  fin_act_0=0
  2nd Order Non-linear Actuator2 : aerolibactuator/Second Order Nonlinear Actuator  SystemSampleTime=-1  wn_fin=wn_act  z_fin=z_act  fin_max=maxdef_rudder  fin_min=mindef_rudder  fin_maxrate=Inf  fin_act_0=0
  Bus Creator : BusCreator  Inputs=3
  Bus Selector1 : BusSelector  OutputSignals=Aileron,Elevator,Rudder
  Positions : Outport
  Sensor_Out : Outport  Port=2
  wires:
  Commands/1 -> Bus Selector1/1
  Bus Selector1/1 -> 2nd Order Non-linear Actuator/1  "<Aileron>"
  Bus Selector1/2 -> 2nd Order Non-linear Actuator1/1  "<Elevator>"
  Bus Selector1/3 -> 2nd Order Non-linear Actuator2/1  "<Rudder>"
  2nd Order Non-linear Actuator2/1 -> Bus Creator/3  "Rudder"
  Bus Creator/1 -> Sensor_Out/1, Positions/1  "Act_positions"
  2nd Order Non-linear Actuator/1 -> Bus Creator/1  "Aileron"
  2nd Order Non-linear Actuator1/1 -> Bus Creator/2  "Elevator"

== system scdskyhogg/Vehicle System Model/Vehicle/Propulsion ==
  cmd : Inport  SampleTime=Ts
  Bus Selector2 : BusSelector  OutputSignals=throttle
  Mux : Mux  Inputs=[1 2]
  ThrustX : Lookup_n-D  NumberOfTableDimensions=1  BreakpointsForDimension1=(1/6)*(3+([-3:3]))  IndexSearchMethod=Linear search  BeginIndexSearchUsingPreviousIndexResult=on  Table=Thrust*(1+tanh([-3:3]))  ExtrapMethod=None - Clip  InputSameDT=on
  Thrust_LMN : Constant  Value=[0, 0, 0]  SampleTime=Ts
  Thrust_YZ : Constant  Value=[0, 0]  SampleTime=Ts
  F : Outport
  M : Outport  Port=2
  wires:
  ThrustX/1 -> Mux/1
  Thrust_YZ/1 -> Mux/2
  Mux/1 -> F/1
  cmd/1 -> Bus Selector2/1
  Thrust_LMN/1 -> M/1
  Bus Selector2/1 -> ThrustX/1  "<throttle>"

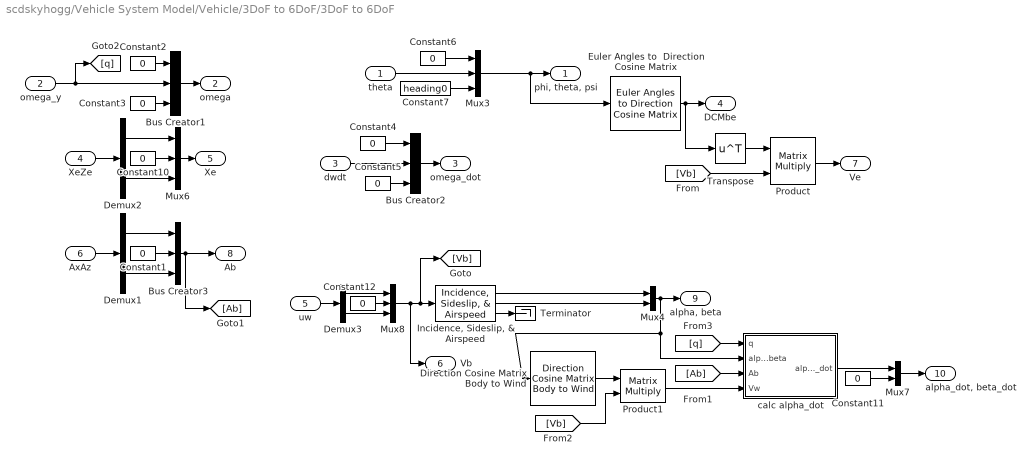
== system scdskyhogg/Vehicle System Model/Vehicle/3DoF to 6DoF/3DoF to 6DoF ==
  theta : Inport
  omega_y : Inport  Port=2
  dwdt : Inport  Port=3
  XeZe : Inport  Port=4
  uw : Inport  Port=5
  AxAz : Inport  Port=6
  Bus Creator1 : BusCreator  Inputs=3
  Bus Creator2 : BusCreator  Inputs=3
  Bus Creator3 : BusCreator  Inputs=3
  Constant{1..6,10..12} (9 alike) : Constant  Value=0
  Constant7 : Constant  Value=heading0
  Demux1 : Demux  Outputs=2
  Demux2 : Demux  Outputs=2
  Demux3 : Demux  Outputs=2
  Direction Cosine Matrix Body to Wind : aerolibtransform2/Direction Cosine Matrix Body to Wind  SystemSampleTime=-1
  Euler Angles to  Direction Cosine Matrix : aerolibobsolete/Euler Angles to  Direction Cosine Matrix  SystemSampleTime=-1
  "Incidence, Sideslip, & Airspeed" : aerolibasang/Incidence, Sideslip, & Airspeed  SystemSampleTime=-1
  Mux3 : Mux  Inputs=3
  Mux4 : Mux  Inputs=2
  Mux6 : Mux  Inputs=3
  Mux7 : Mux  Inputs=2
  Mux8 : Mux  Inputs=3
  Product : Product  Multiplication=Matrix(*)  SaturateOnIntegerOverflow=on  InputSameDT=on  OutDataTypeStr=Inherit: Same as first input
  Product1 : Product  Multiplication=Matrix(*)  SaturateOnIntegerOverflow=on  InputSameDT=on  OutDataTypeStr=Inherit: Same as first input
  Terminator : Terminator
  Transpose : Math  Operator=transpose  SaturateOnIntegerOverflow=on
  calc alpha_dot : Subsystem
  "phi, theta, psi" : Outport
  omega : Outport  Port=2
  omega_dot : Outport  Port=3
  DCMbe : Outport  Port=4
  Xe : Outport  Port=5
  Vb : Outport  Port=6
  Ve : Outport  Port=7
  Ab : Outport  Port=8
  "alpha, beta" : Outport  Port=9
  "alpha_dot, beta_dot" : Outport  Port=10
  wires:
  omega_y/1 -> Bus Creator1/2, [q]
  Bus Creator3/1 -> [Ab], Ab/1
  Demux1/1 -> Bus Creator3/1
  Demux1/2 -> Bus Creator3/3
  Constant1/1 -> Bus Creator3/2
  Constant2/1 -> Bus Creator1/1
  Constant3/1 -> Bus Creator1/3
  Constant4/1 -> Bus Creator2/1
  Constant5/1 -> Bus Creator2/3
  Constant6/1 -> Mux3/1
  Constant7/1 -> Mux3/3
  Mux3/1 -> Euler Angles to  Direction Cosine Matrix/1, "phi, theta, psi"/1
  Mux4/1 -> calc alpha_dot/2(alpha,beta), Direction Cosine Matrix Body to Wind/1, "alpha, beta"/1
  "Incidence, Sideslip, & Airspeed"/2 -> Mux4/2
  Demux2/1 -> Mux6/1
  Demux2/2 -> Mux6/3
  Constant10/1 -> Mux6/2
  Transpose/1 -> Product/1
  [Vb] -> Product/2
  calc alpha_dot/1(alpha_dot) -> Mux7/1
  [Ab] -> calc alpha_dot/3(Ab)
  [Vb] -> Product1/2
  [q] -> calc alpha_dot/1(q)
  Constant11/1 -> Mux7/2
  Demux3/2 -> Mux8/3
  Constant12/1 -> Mux8/2
  Demux3/1 -> Mux8/1
  Direction Cosine Matrix Body to Wind/1 -> Product1/1
  Product1/1 -> calc alpha_dot/4(Vw)
  "Incidence, Sideslip, & Airspeed"/1 -> Mux4/1
  "Incidence, Sideslip, & Airspeed"/3 -> Terminator/1
  theta/1 -> Mux3/2
  Bus Creator1/1 -> omega/1
  dwdt/1 -> Bus Creator2/2
  Bus Creator2/1 -> omega_dot/1
  XeZe/1 -> Demux2/1
  Mux6/1 -> Xe/1
  uw/1 -> Demux3/1
  AxAz/1 -> Demux1/1
  Product/1 -> Ve/1
  Mux7/1 -> "alpha_dot, beta_dot"/1
  Mux8/1 -> "Incidence, Sideslip, & Airspeed"/1, [Vb], Vb/1
  Euler Angles to  Direction Cosine Matrix/1 -> DCMbe/1, Transpose/1

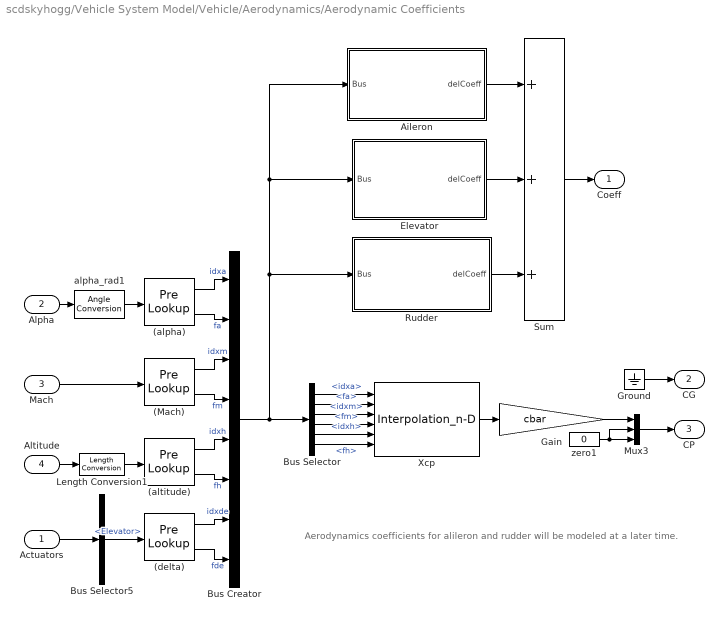
== system scdskyhogg/Vehicle System Model/Vehicle/Aerodynamics/Aerodynamic Coefficients ==
  note: Aerodynamics coefficients for alileron and rudder will be modeled at a later time.
  Actuators : Inport
  Alpha : Inport  Port=2
  Mach : Inport  Port=3
  Altitude : Inport  Port=4
  (Mach) : PreLookup  BreakpointsData=statdyn{1}.mach  BeginIndexSearchUsingPreviousIndexResult=on  ProcessOutOfRangeInput=Linear extrapolation  IndexDataTypeStr=int32  FractionDataTypeStr=double
  (alpha) : PreLookup  BreakpointsData=statdyn{1}.alpha  BeginIndexSearchUsingPreviousIndexResult=on  ProcessOutOfRangeInput=Linear extrapolation  IndexDataTypeStr=int32  FractionDataTypeStr=double
  (altitude) : PreLookup  BreakpointsData=statdyn{1}.alt  BeginIndexSearchUsingPreviousIndexResult=on  ProcessOutOfRangeInput=Linear extrapolation  IndexDataTypeStr=int32  FractionDataTypeStr=double
  (delta) : PreLookup  BreakpointsData=statdyn{1}.delta  BeginIndexSearchUsingPreviousIndexResult=on  ProcessOutOfRangeInput=Linear extrapolation  IndexDataTypeStr=int32  FractionDataTypeStr=double
  Aileron : Subsystem
  Bus Creator : BusCreator  Inputs=8
  Bus Selector : BusSelector  OutputSignals=idxa,fa,idxm,fm,idxh,fh
  Bus Selector5 : BusSelector  OutputSignals=Elevator
  Elevator : Subsystem
  Gain : Gain  Gain=cbar
  Ground : Ground
  Length Conversion1 : aerolibconvert2/Length Conversion  SystemSampleTime=-1  IU=m  OU=ft
  Mux3 : Mux  Inputs=3
  Rudder : Subsystem
  Sum : Sum  Inputs=3  SaturateOnIntegerOverflow=on  InputSameDT=on  OutDataTypeStr=Inherit: Same as first input
  Xcp : Interpolation_n-D  NumberOfTableDimensions=3  Table="permute(statdyn{1}.xcp,[1  2  3])"  OutDataTypeStr=double
      settings: InputPortMap=u0,u1,u2,u3,u4,u5
  alpha_rad1 : aerolibconvert2/Angle Conversion  SystemSampleTime=-1  IU=rad  OU=deg
  zero1 : Constant  Value=0
  Coeff : Outport  InitialOutput=0
  CG : Outport  Port=2  PortDimensions=3  InitialOutput=0
  CP : Outport  Port=3  PortDimensions=3  InitialOutput=0
  wires:
  Sum/1 -> Coeff/1
  Actuators/1 -> Bus Selector5/1
  Ground/1 -> CG/1
  Mux3/1 -> CP/1
  Xcp/1 -> Gain/1
  zero1/1 -> Mux3/2, Mux3/3
  Gain/1 -> Mux3/1
  (alpha)/2 -> Bus Creator/2  "fa"
  (Mach)/2 -> Bus Creator/4  "fm"
  (altitude)/2 -> Bus Creator/6  "fh"
  (altitude)/1 -> Bus Creator/5  "idxh"
  (Mach)/1 -> Bus Creator/3  "idxm"
  (alpha)/1 -> Bus Creator/1  "idxa"
  Bus Selector/1 -> Xcp/1  "<idxa>"
  Bus Selector/2 -> Xcp/2  "<fa>"
  Bus Selector/3 -> Xcp/3  "<idxm>"
  Bus Selector/4 -> Xcp/4  "<fm>"
  Bus Selector/5 -> Xcp/5  "<idxh>"
  Bus Selector/6 -> Xcp/6  "<fh>"
  Bus Creator/1 -> Bus Selector/1, Elevator/1(Bus), Aileron/1(Bus), Rudder/1(Bus)
  Mach/1 -> (Mach)/1
  Altitude/1 -> Length Conversion1/1
  Length Conversion1/1 -> (altitude)/1
  Alpha/1 -> alpha_rad1/1
  alpha_rad1/1 -> (alpha)/1
  Aileron/1(delCoeff) -> Sum/1
  Elevator/1(delCoeff) -> Sum/2
  Rudder/1(delCoeff) -> Sum/3
  (delta)/1 -> Bus Creator/7  "idxde"
  (delta)/2 -> Bus Creator/8  "fde"
  Bus Selector5/1 -> (delta)/1  "<Elevator>"

== system scdskyhogg/Vehicle System Model/Vehicle/Aerodynamics/DerivedConditions ==
  Speed of Sound : Inport
  Air Density : Inport  Port=2
  WindVelocity : Inport  Port=3  PortDimensions=3
  WindAngularRates : Inport  Port=4  PortDimensions=3
  Vb : Inport  Port=5  PortDimensions=3
  Dynamic Pressure : aerolibasang/Dynamic Pressure  SystemSampleTime=-1
  Mach Number : aerolibasang/Mach Number  SystemSampleTime=-1
  Sum2 : Sum  Inputs=|+-  SaturateOnIntegerOverflow=on  InputSameDT=on  OutDataTypeStr=Inherit: Same as first input
  Mach : Outport
  qbar : Outport  Port=2  InitialOutput=0
  "pqrWind " : Outport  Port=3
  wires:
  Speed of Sound/1 -> Mach Number/2
  Mach Number/1 -> Mach/1  "Mach"
  Air Density/1 -> Dynamic Pressure/2
  Dynamic Pressure/1 -> qbar/1  "qbar"
  WindAngularRates/1 -> "pqrWind "/1
  Vb/1 -> Sum2/1
  Sum2/1 -> Dynamic Pressure/1, Mach Number/1
  WindVelocity/1 -> Sum2/2

== system scdskyhogg/Vehicle System Model/Vehicle/3DoF to 6DoF/3DoF to 6DoF/calc alpha_dot ==
  q : Inport
  alpha,beta : Inport  Port=2
  Ab : Inport  Port=3
  Vw : Inport  Port=4
  Direction Cosine Matrix Body to Wind : aerolibtransform2/Direction Cosine Matrix Body to Wind  SystemSampleTime=-1
  Product1 : Product  Multiplication=Matrix(*)  SaturateOnIntegerOverflow=on  InputSameDT=on  OutDataTypeStr=Inherit: Same as first input
  Product2 : Product  Inputs=*/  SaturateOnIntegerOverflow=on  InputSameDT=on  OutDataTypeStr=Inherit: Same as first input
  Selector2 : Selector  InputPortWidth=3  IndexOptions=Index vector (dialog)  Indices=3  OutputSizes=1
  Selector3 : Selector  InputPortWidth=3  IndexOptions=Index vector (dialog)  Indices=1  OutputSizes=1
  Sum : Sum  Inputs=++|
  Transpose1 : Math  Operator=transpose  SaturateOnIntegerOverflow=on
  alpha_dot : Outport
  wires:
  Direction Cosine Matrix Body to Wind/1 -> Transpose1/1
  Transpose1/1 -> Product1/1
  Product1/1 -> Selector2/1
  Selector2/1 -> Product2/1
  Selector3/1 -> Product2/2
  Product2/1 -> Sum/2
  alpha,beta/1 -> Direction Cosine Matrix Body to Wind/1
  q/1 -> Sum/1
  Sum/1 -> alpha_dot/1
  Ab/1 -> Product1/2
  Vw/1 -> Selector3/1

== system scdskyhogg/Vehicle System Model/Vehicle/Aerodynamics/Aerodynamic Coefficients/Aileron ==
  note: Aerodynamics coefficients for alileron and rudder will be modeled at a later time when 6DOF model is developed.
  Bus : Inport
  Constant1 : Constant  Value=0
  Mux1 : Mux  Inputs=6
  Terminator : Terminator
  delCoeff : Outport
  wires:
  Mux1/1 -> delCoeff/1
  Constant1/1 -> Mux1/1, Mux1/2, Mux1/3, Mux1/4, Mux1/5, Mux1/6
  Bus/1 -> Terminator/1

== system scdskyhogg/Vehicle System Model/Vehicle/Aerodynamics/Aerodynamic Coefficients/Elevator ==
  Bus : Inport
  Bus Selector2 : BusSelector  OutputSignals=idxa,fa,idxm,fm,idxh,fh,idxde,fde
  Bus Selector3 : BusSelector  OutputSignals=idxde,fde,idxm,fm,idxh,fh
  Bus Selector5 : BusSelector  OutputSignals=idxde,fde,idxm,fm,idxh,fh
  Constant1 : Constant  Value=0
  DCDI : Interpolation_n-D  NumberOfTableDimensions=4  Table=permute(statdyn{1}.dcdi_sym,[1 3 4 2 ])  CheckIndexInCode=off
      settings: InputPortMap=u0,u1,u2,u3,u4,u5,u6,u7
  DCL : Interpolation_n-D  NumberOfTableDimensions=3  Table="permute(statdyn{1}.dcl_sym,[1  2  3])"  CheckIndexInCode=off
      settings: InputPortMap=u0,u1,u2,u3,u4,u5
  DCm : Interpolation_n-D  NumberOfTableDimensions=3  Table="permute(statdyn{1}.dcm_sym,[1  2  3])"  CheckIndexInCode=off
      settings: InputPortMap=u0,u1,u2,u3,u4,u5
  Mux1 : Mux  Inputs=6
  delCoeff : Outport
  wires:
  Mux1/1 -> delCoeff/1
  Bus/1 -> Bus Selector2/1, Bus Selector3/1, Bus Selector5/1
  DCDI/1 -> Mux1/1
  DCL/1 -> Mux1/3
  DCm/1 -> Mux1/5
  Constant1/1 -> Mux1/2, Mux1/4, Mux1/6
  Bus Selector2/1 -> DCDI/1  "<idxa>"
  Bus Selector2/2 -> DCDI/2  "<fa>"
  Bus Selector3/1 -> DCL/1  "<idxde>"
  Bus Selector3/2 -> DCL/2  "<fde>"
  Bus Selector5/1 -> DCm/1  "<idxde>"
  Bus Selector5/2 -> DCm/2  "<fde>"
  Bus Selector2/3 -> DCDI/3  "<idxm>"
  Bus Selector2/4 -> DCDI/4  "<fm>"
  Bus Selector2/5 -> DCDI/5  "<idxh>"
  Bus Selector2/6 -> DCDI/6  "<fh>"
  Bus Selector2/7 -> DCDI/7  "<idxde>"
  Bus Selector2/8 -> DCDI/8  "<fde>"
  Bus Selector3/3 -> DCL/3  "<idxm>"
  Bus Selector3/4 -> DCL/4  "<fm>"
  Bus Selector3/5 -> DCL/5  "<idxh>"
  Bus Selector3/6 -> DCL/6  "<fh>"
  Bus Selector5/3 -> DCm/3  "<idxm>"
  Bus Selector5/4 -> DCm/4  "<fm>"
  Bus Selector5/5 -> DCm/5  "<idxh>"
  Bus Selector5/6 -> DCm/6  "<fh>"

== system scdskyhogg/Vehicle System Model/Vehicle/Aerodynamics/Aerodynamic Coefficients/Rudder ==
  note: Aerodynamics coefficients for alileron and rudder will be modeled at a later time when 6DOF model is developed.
  Bus : Inport
  Constant1 : Constant  Value=0
  Mux1 : Mux  Inputs=6
  Terminator : Terminator
  delCoeff : Outport
  wires:
  Mux1/1 -> delCoeff/1
  Constant1/1 -> Mux1/6, Mux1/5, Mux1/4, Mux1/3, Mux1/2, Mux1/1
  Bus/1 -> Terminator/1
